simulink model "HILModel"  (R2016a)
settings: Solver=ode23tb  StartTime=0.0  StopTime=1000  RelTol=1e-3
libraries: DAEMOT_Lib x52
settings Model: Creator=aksland2  LastModifiedBy=aksland2

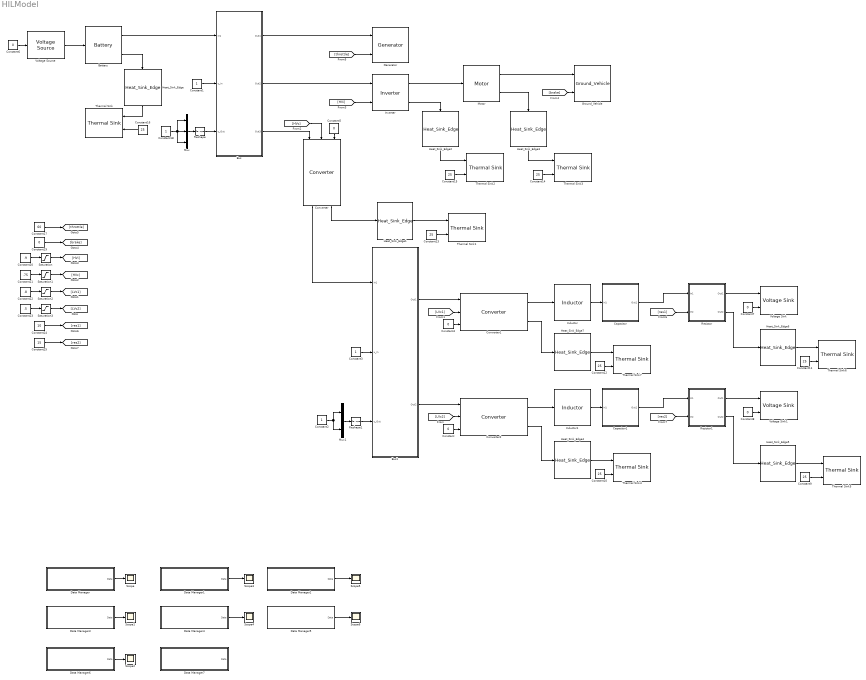
== system HILModel ==
  Battery : DAEMOT_Lib/Dyn Electrical Comp/Battery  C_c=62.7  C_s=4.5  R_cond=1.94  B_cap=5.088600000000000  Ns=16  Np=1  batt=4.2V LiPo 5.1 Ah  Ts_initial=25  Tc_initial=25  SOC_initial=.9  RC_initial=[0 0]
  Bus : Subsystem  AncestorBlock=DAEMOT_Lib/Electrical Components Chris/Bus  mask{R=.1, L=.0001, C=1, Num_In=1, Num_Out=3, V_initial=.5, I_initial=0}
      mask prompts: R "Resistance [Ohm]"; L "Inductance [H]"; C "Capacitance [F]"; Num_In "Number of Inputs"; Num_Out "Number of Outputs"; V_initial "Initial Voltage [V]"; I_initial "Initial Current [A]"
      mask init:
      | h      = get_param(gcb,'handle');   % Get block handle
      | blk    = gcb;
      | hblock = get(h);     % Parse out handles structure
      | 
      | %%%%%%%%%%%%%%%%%%%%%%%%%%%%%% Clear Stuff %%%%%%%%%%%%%%%%%%%%%%%%%%%%%%%%
      | %delete any previous inports and bus selectors
      | for i = str2num(hblock.Num_In)+1:hblock.Ports(1)-2
      |     delete_block([blk,'/In',num2str(i)])
      |     delete_block([blk,'/gb',num2str(i)])
      |     delete_block([blk,'/vm',num2str(i)])
      |     delete_block([blk,'/term',num2str(i)])
      |     delete_block([blk,'/Sink',num2str(i)])
      |     delete_block([blk,'/vin',num2str(i)])
      |     
      |     delete_unconnected_lines(blk)
      | end
      | 
      | for i = str2num(hblock.Num_Out)+1:hblock.Ports(2)
      |     delete_block([blk,'/Out',num2str(i)])
      |     delete_block([blk,'/if',num2str(i)])
      |     delete_block([blk,'/io',num2str(i)])
      |     delete_block([blk,'/vo',num2str(i)])
      |     delete_block([blk,'/vot',num2str(i)])
      |     delete_block([blk,'/b',num2str(i)])
      |     delete_block([blk,'/Source',num2str(i)])
      |     delete_block([blk,'/ig',num2str(i)])
      |     delete_block([blk,'/ios',num2str(i)])
      |     
      |     delete_unconnected_lines(blk)
      | end
      | %%%%%%%%%%%%%%%%%%%%%%%%%%%%% Clear Stuff %%%%%%%%%%%%%%%%%%%%%%%%%%%%%%%%
      | 
      | %%%%%%%%%%%%%%%%%%%%%%%%%%%%%% Edit Mux inputs %%%%%%%%%%%%%%%%%%%%%%%%%%%%%%%%
      | set_param([blk,'/Mux_In_1'],'Inputs',hblock.Num_In)
      | set_param([blk,'/Mux_In_2'],'Inputs',hblock.Num_Out)
      | set_param([blk,'/Demux_Out_1'],'Outputs',hblock.Num_In)
      | set_param([blk,'/Demux_Out_2'],'Outputs',hblock.Num_Out)
      | set_param([blk,'/u_Out'],'Port',num2str(Num_In+2))
      | set_param([blk,'/u_In'],'Port',num2str(Num_In+1))
      | set_param([blk,'/Bus_Sink_1'],'Inputs',num2str(str2num(hblock.Num_Out)+1))
      | 
      | %%%%%%%%%%%%%%%%%%%%%%%%%%%%%% Edit Mux inputs %%%%%%%%%%%%%%%%%%%%%%%%%%%%%%%%
      | 
      | %%%%%%%%%%%%%%%%%%%%%%%%%%%%%% Create and Place Inputs %%%%%%%%%%%%%%%%%%%%%%%%%%%%%%%%
      | % generate inports, bus selectors, and route lines to each vector concat
      | for i = hblock.Ports(1)+1-2:str2num(hblock.Num_In)
      |     
      |     % add blocks (positioning notation [x i*s+y x+l i*s+h+y] x:(horiz. pos.), y:(vert. pos.), s:(spacing), l:(horiz. length), x:(vert. height)
      |     add_block('simulink/Ports & Subsystems/In1',   [blk,'/In',num2str(i)],    'Position',[355 i*80+425 355+30 i*80+13+425]);         % adding inport
      |     add_block([blk,'/gb1'],                        [blk,'/gb',num2str(i)],   'Position',[440 i*80+410 440+5 i*80+38+410]);         % adding inport
      |     add_block('simulink/Signal Routing/Goto',      [blk,'/vm',num2str(i)],    'Position',[500 i*80+450 500+80 i*80+14+450]);         % adding inport
      |     add_block('simulink/Sinks/Terminator',          [blk,'/term',num2str(i)],    'Position',[500 i*80+415 500+20 i*80+14+415]);         % adding inport
      |     add_block('DAEMOT_Lib/Support Functions/Sink',[blk,'/Sink',num2str(i)],'Position',[200 i*30+336 200+65 i*30+28+336]);         % adding inport
      |     add_block('simulink/Signal Routing/From',       [blk,'/vin',num2str(i)],     'Position',[-400 i*20+405 -400+80 i*20+18+405]);         % adding inport
      |     
      |     % set goto and from tags
      |     set_param([blk,'/vm',num2str(i)],'GotoTag',char(horzcat('V_in',num2str(i))))
      |     set_param([blk,'/vin',num2str(i)],'GotoTag',char(horzcat('V_in',num2str(i))))
      |     
      |     % set goto and from background colors
      | %    set_param([blk,'/gm',num2str(i)],'BackgroundColor','yellow')
      | %    set_param([blk,'/gt',num2str(i)],'BackgroundColor','yellow')
      | %    %set_param([blk,'/gp',num2str(i)],'BackgroundColor','yellow')
      | %    set_param([blk,'/min',num2str(i)],'BackgroundColor','yellow')
      | %    set_param([blk,'/tin',num2str(i)],'BackgroundColor','yellow')
      | %    set_param([blk,'/pout',num2str(i)],'BackgroundColor','cyan')
      |     
      |     % add lines
      |     add_line(blk,['In',num2str(i),'/1'], ['gb',num2str(i),'/1'],'AutoRouting','on')
      |     add_line(blk,['gb',num2str(i),'/2'],  ['vm',num2str(i),'/1'],'AutoRouting','on')
      |     add_line(blk,['gb',num2str(i),'/1'],  ['term',num2str(i),'/1'],'AutoRouting','on')
      |     add_line(blk,['Demux_Out_1/',num2str(i)],  ['Sink',num2str(i),'/1'],'AutoRouting','on')
      |     add_line(blk,['vin',num2str(i),'/1'],  ['Mux_In_1/',num2str(i)],'AutoRouting','on')
      | %     
      | end
      | %%%%%%%%%%%%%%%%%%%%%%%%%%%%%% Create and Place Inputs %%%%%%%%%%%%%%%%%%%%%%%%%%%%%%%%
      | 
      | %%%%%%%%%%%%%%%%%%%%%%%%%%%%%% Create and Place Outputs %%%%%%%%%%%%%%%%%%%%%%%%%%%%%%%%
      | % generate inports, bus selectors, and route lines to each vector concat
      | for i = hblock.Ports(2)+1:str2num(hblock.Num_Out)
      |     
      |     % add blocks
      |     add_block('simulink/Ports & Subsystems/Out1',   [blk,'/Out',num2str(i)],   'Position',[875 i*80+425 875+30 i*80+13+425]);         % adding inport
      |     add_block('simulink/Signal Routing/Bus Creator',[blk,'/b',num2str(i)],     'Position',[825 i*80+410 825+5 i*80+38+410]);         % adding inport
      |     add_block('simulink/Signal Routing/From',       [blk,'/io',num2str(i)],     'Position',[710 i*80+415 710+80 i*80+14+415]);         % adding inport
      |     add_block('simulink/Signal Routing/From',       [blk,'/vo',num2str(i)],     'Position',[710 i*80+435 710+80 i*80+14+435]);         % adding inport
      |     add_block('simulink/Signal Routing/Goto',       [blk,'/vot',num2str(i)],     'Position',[1250 i*20+50 1250+80 i*20+18+50]);         % adding inport
      |     add_block('simulink/Signal Routing/From',       [blk,'/if',num2str(i)],     'Position',[935 i*20+410 935+80 i*20+18+410]);         % adding inport
      |     add_block('DAEMOT_Lib/Support Functions/Source',[blk,'/Source',num2str(i)],'Position',[1400 i*30+420 1400+65 i*30+28+420]);         % adding inport
      |     add_block('simulink/Signal Routing/Goto',       [blk,'/ig',num2str(i)],     'Position',[1550 i*30+430 1550+80 i*30+14+430]);         % adding inport
      |     add_block('simulink/Signal Routing/From',       [blk,'/ios',num2str(i)],     'Position',[1770 i*16+405 1770+80 i*16+14+405]);         % adding inport
      |     
      |     % set goto and from tags
      |     set_param([blk,'/if',num2str(i)],'GotoTag',char(horzcat('I_out',num2str(i))))
      |     set_param([blk,'/io',num2str(i)],'GotoTag',char(horzcat('I_out',num2str(i))))
      |     set_param([blk,'/vo',num2str(i)],'GotoTag',char(horzcat('V_out',num2str(i))))
      |     set_param([blk,'/vot',num2str(i)],'GotoTag',char(horzcat('V_out',num2str(i))))
      |     set_param([blk,'/ig',num2str(i)],'GotoTag',char(horzcat('I_out',num2str(i))))
      |     set_param([blk,'/ios',num2str(i)],'GotoTag',char(horzcat('I_out',num2str(i))))
      |     set_param([blk,'/b',num2str(i)],'Inputs','2')
      |     
      | %     % set goto and from background colors
      | %     set_param([blk,'/t',num2str(i)],'BackgroundColor','cyan')
      | %     set_param([blk,'/m',num2str(i)],'BackgroundColor','cyan')
      | %     set_param([blk,'/p',num2str(i)],'BackgroundColor','cyan')
      | %     set_param([blk,'/g',num2str(i)],'BackgroundColor','cyan')
      | %     set_param([blk,'/mout',num2str(i)],'BackgroundColor','cyan')
      | %     %set_param([blk,'/tout',num2str(i)],'BackgroundColor','cyan')
      |     
      |     % add lines
      |     add_line(blk,['io',num2str(i),'/1'],['b',num2str(i),'/1'],'AutoRouting','on')
      |     p = get_param([blk,'/io',num2str(i)],'PortHandles');
      |     l = get_param(p.Outport,'Line');
      |     set_param(l,'Name','current')
      |     
      |     add_line(blk,['vo',num2str(i),'/1'],['b',num2str(i),'/2'],'AutoRouting','on')
      |     p = get_param([blk,'/vo',num2str(i)],'PortHandles');
      |     l = get_param(p.Outport,'Line');
      |     set_param(l,'Name','voltage')
      |         
      |     add_line(blk,['ios',num2str(i),'/1'],['Bus_Sink_1/',num2str(i+1)],'AutoRouting','on')
      |     p = get_param([blk,'/ios',num2str(i)],'PortHandles');
      |     l = get_param(p.Outport,'Line');
      |     set_param(l,'Name',['Current',num2str(i)])
      |      
      |     add_line(blk,['b',num2str(i),'/1'],['Out',num2str(i),'/1'],'AutoRouting','on')
      |     add_line(blk,['Source',num2str(i),'/1'],['ig',num2str(i),'/1'],'AutoRouting','on')
      |     add_line(blk,['if',num2str(i),'/1'],  ['Mux_In_2/',num2str(i)],'AutoRouting','on')
      |     add_line(blk,['Demux_Out_2/',num2str(i)],['vot',num2str(i),'/1'],'AutoRouting','on')
      |     
      | 
      | 
      | end
      | %%%%%%%%%%%%%%%%%%%%%%%%%%%%%% Create and Place Outputs %%%%%%%%%%%%%%%%%%%%%%%%%%%%%%%%
      | 
      | try
      |     set_param([blk,'/Selector1'],'InputPortWidth',num2str(hblock.Num_In))
      |     
      |     selector_str = '[1 ';
      |     for i = 2:str2num(hblock.Num_In)
      |         selector_str = [selector_str,num2str(i),' '];
      |     end
      |     selector_str = [selector_str,']'];
      |     set_param([blk,'/Selector1'],'IndexParamArray',{selector_str})%num2cell(1:hblock.Num_In))
      | catch
      |     selector_str = '[1 ';
      |     for i = 2:str2num(hblock.Num_In)
      |         selector_str = [selector_str,num2str(i),' '];
      |     end
      |     selector_str = [selector_str,']'];
      |     set_param([blk,'/Selector1'],'IndexParamArray',{selector_str})%num2cell(1:hblock.Num_In))
      |     
      |     set_param([blk,'/Selector1'],'InputPortWidth',num2str(hblock.Num_In))
      | end 
      |     
      | try
      |     set_param([blk,'/Selector2'],'InputPortWidth',num2str(hblock.Num_Out))
      |     
      |     selector_str = '[1 ';
      |     for i = 2:str2num(hblock.Num_Out)
      |         selector_str = [selector_str,num2str(i),' '];
      |     end
      |     selector_str = [selector_str,']'];
      |     set_param([blk,'/Selector2'],'IndexParamArray',{selector_str})%num2cell(1:hblock.Num_Out))
      | catch
      |     selector_str = '[1 ';
      |     for i = 2:str2num(hblock.Num_Out)
      |         selector_str = [selector_str,num2str(i),' '];
      |     end
      |     selector_str = [selector_str,']'];
      |     set_param([blk,'/Selector2'],'IndexParamArray',{selector_str})%num2cell(1:hblock.Num_Out))
      |     
      |     set_param([blk,'/Selector2'],'InputPortWidth',num2str(hblock.Num_Out))
      | end 
      | 
      |     clear h blk hblock
      settings: CopyFcn=|
      | h      = get_param(gcb,'handle');   % Get block handle
      | blk    = gcb;
      | 
      | set_param(blk, 'LinkStatus', 'inactive')
      | clear h
      | clear blk
      mask Display:
      | text(0.5,0.95,['{\bf Bus}'],'TexMode','on','horizontalAlignment', 'center')
      | text(0.5,0.075,['{\bf ----(V)}'],'TexMode','on','horizontalAlignment', 'center')
      | 
      | In = get_param(gcb,'Num_In');
      | Out = get_param(gcb,'Num_Out');
      | 
      | for i = 1:str2num(In)
      |     port_label('input',i,['Electrical In ',num2str(i)])
      | end
      | 
      | port_label('input',str2num(In)+1,'u_In')
      | port_label('input',str2num(In)+2,'u_Out')
      | 
      | for i = 1:str2num(Out)
      |     port_label('output',i,['Electrical Out ',num2str(i)])
      | end
  Bus1 : Subsystem  AncestorBlock=DAEMOT_Lib/Electrical Components Chris/Bus  mask{R=.1, L=.0001, C=1, Num_In=1, Num_Out=2, V_initial=.5, I_initial=0}
      mask prompts: R "Resistance [Ohm]"; L "Inductance [H]"; C "Capacitance [F]"; Num_In "Number of Inputs"; Num_Out "Number of Outputs"; V_initial "Initial Voltage [V]"; I_initial "Initial Current [A]"
      mask init: same as HILModel/Bus
      settings: CopyFcn=|
      | h      = get_param(gcb,'handle');   % Get block handle
      | blk    = gcb;
      | 
      | set_param(blk, 'LinkStatus', 'inactive')
      | clear h
      | clear blk
      mask Display:
      | text(0.5,0.95,['{\bf Bus}'],'TexMode','on','horizontalAlignment', 'center')
      | text(0.5,0.075,['{\bf ----(V)}'],'TexMode','on','horizontalAlignment', 'center')
      | 
      | In = get_param(gcb,'Num_In');
      | Out = get_param(gcb,'Num_Out');
      | 
      | for i = 1:str2num(In)
      |     port_label('input',i,['Electrical In ',num2str(i)])
      | end
      | 
      | port_label('input',str2num(In)+1,'u_In')
      | port_label('input',str2num(In)+2,'u_Out')
      | 
      | for i = 1:str2num(Out)
      |     port_label('output',i,['Electrical Out ',num2str(i)])
      | end
  Capacitor : Subsystem  AncestorBlock=DAEMOT_Lib/Electrical Components Chris/Capacitor  mask{C=3, V_initial=0}
      mask prompts: C "Capacitance [F]"; V_initial "Initial Ouput Voltage [V]"
      mask init:
      | % if strcmp(Gn_check,'off')
      | %     %is not ground node
      | %     Gn = 0;
      | %     %V_initial = V_initial_temp;
      | % else
      | %     %is ground node
      | %     Gn = 1;
      | %     %V_initial = 0;
      | % end
      mask Display:
      | image(imread('capacitor.bmp'));
      | text(0.5,0.95,['{\bf Capacitor}'],'TexMode','on','horizontalAlignment', 'center')
      | text(0.5,0.075,['{\bf (V)}'],'TexMode','on','horizontalAlignment', 'center')
      | 
      | port_label('input',1,sprintf('Electrical \nIn'))
      | %port_label('input',2,'Capacitance')
      | port_label('output',1,sprintf('Electrical \nOut'))
  Capacitor1 : Subsystem  AncestorBlock=DAEMOT_Lib/Electrical Components Chris/Capacitor  mask{C=3, V_initial=0}
      mask prompts: C "Capacitance [F]"; V_initial "Initial Ouput Voltage [V]"
      mask init:
      | % if strcmp(Gn_check,'off')
      | %     %is not ground node
      | %     Gn = 0;
      | %     %V_initial = V_initial_temp;
      | % else
      | %     %is ground node
      | %     Gn = 1;
      | %     %V_initial = 0;
      | % end
      mask Display:
      | image(imread('capacitor.bmp'));
      | text(0.5,0.95,['{\bf Capacitor}'],'TexMode','on','horizontalAlignment', 'center')
      | text(0.5,0.075,['{\bf (V)}'],'TexMode','on','horizontalAlignment', 'center')
      | 
      | port_label('input',1,sprintf('Electrical \nIn'))
      | %port_label('input',2,'Capacitance')
      | port_label('output',1,sprintf('Electrical \nOut'))
  Constant{,4..8,19} (7 alike) : Constant  Value=0
  Constant{1..3,18} (4 alike) : Constant
  Constant{9..16} (8 alike) : Constant  Value=25
  Constant17 : Constant  Value=60
  Constant20 : Constant  Value=.9
  Constant21 : Constant  Value=.75
  Constant22 : Constant  Value=.8
  Constant23 : Constant  Value=.5
  Constant24 : Constant  Value=10
  Constant25 : Constant  Value=15
  Converter : DAEMOT_Lib/Dyn Electrical Comp/Converter  V_D=.01  R_D=.01  R_s=.01  R_L=.01  dir=<===  Cp=60  T_initial=25
  Converter1 : DAEMOT_Lib/Dyn Electrical Comp/Converter  V_D=.01  R_D=.01  R_s=.01  R_L=.01  dir=<===  Cp=60  T_initial=25
  Converter2 : DAEMOT_Lib/Dyn Electrical Comp/Converter  V_D=.01  R_D=.01  R_s=.01  R_L=.01  dir=<===  Cp=60  T_initial=25
  Data Manager : Subsystem  AncestorBlock=DAEMOT_Lib/Support Functions/Data Manager  mask{null=0}
      mask init:
      | set_param(gcb, 'LinkStatus', 'inactive')    % disable the library link
      settings: OpenFcn=data_manager
      mask Display: str ='Battery/SOC'; fprintf(str)
  Data Manager1 : Subsystem  AncestorBlock=DAEMOT_Lib/Support Functions/Data Manager  mask{null=0}
      mask init:
      | set_param(gcb, 'LinkStatus', 'inactive')    % disable the library link
      settings: OpenFcn=data_manager
      mask Display: str ='Bus/Voltage'; fprintf(str)
  Data Manager2 : Subsystem  AncestorBlock=DAEMOT_Lib/Support Functions/Data Manager  mask{null=0}
      mask init:
      | set_param(gcb, 'LinkStatus', 'inactive')    % disable the library link
      settings: OpenFcn=data_manager
      mask Display: str ='Bus1/Voltage'; fprintf(str)
  Data Manager3 : Subsystem  AncestorBlock=DAEMOT_Lib/Support Functions/Data Manager  mask{null=0}
      mask init:
      | set_param(gcb, 'LinkStatus', 'inactive')    % disable the library link
      settings: OpenFcn=data_manager
      mask Display: str ='Motor/Speed'; fprintf(str)
  Data Manager4 : Subsystem  AncestorBlock=DAEMOT_Lib/Support Functions/Data Manager  mask{null=0}
      mask init:
      | set_param(gcb, 'LinkStatus', 'inactive')    % disable the library link
      settings: OpenFcn=data_manager
      mask Display: str ='Ground_Vehicle/Vehicle Speed'; fprintf(str)
  Data Manager5 : Subsystem  AncestorBlock=DAEMOT_Lib/Support Functions/Data Manager  mask{null=0}
      mask init:
      | set_param(gcb, 'LinkStatus', 'inactive')    % disable the library link
      settings: OpenFcn=data_manager
      mask Display: str ='Generator/Current'; fprintf(str)
  Data Manager6 : Subsystem  AncestorBlock=DAEMOT_Lib/Support Functions/Data Manager  mask{null=0}
      mask init:
      | set_param(gcb, 'LinkStatus', 'inactive')    % disable the library link
      settings: OpenFcn=data_manager
      mask Display: str ='Resistor/Current\nResistor1/Current'; fprintf(str)
  Data Manager7 : Subsystem  AncestorBlock=DAEMOT_Lib/Support Functions/Data Manager  mask{null=0}
      mask init:
      | set_param(gcb, 'LinkStatus', 'inactive')    % disable the library link
      settings: OpenFcn=data_manager
      mask Display: str ='Ground_Vehicle/Vehicle Speed'; fprintf(str)
  Generator : DAEMOT_Lib/Dyn Electrical Comp/Generator  G=1
  Ground_Vehicle : DAEMOT_Lib/Dyn Electrical Comp/Ground_Vehicle  R=.3  Af=2  rho_air=1.2  Cd=.26
  Heat_Sink_Edge{,1..7} (8 alike) : DAEMOT_Lib/Dyn Electrical Comp/Heat_Sink_Edge  s=off  R_const=1  k=237  As=.025  L=.02
  Inductor : DAEMOT_Lib/Dyn Electrical Comp/Inductor  L=.0001  I_initial=0
  Inductor1 : DAEMOT_Lib/Dyn Electrical Comp/Inductor  L=.0001  I_initial=0
  Inverter : DAEMOT_Lib/Dyn Electrical Comp/Inverter  R1=.01  R2=.01  R3=.01  Cp=60  T_initial=25
  Motor : DAEMOT_Lib/Dyn Electrical Comp/Motor  R=0.013461960749493  L=1.252192537082724e-05  Kv=0.009688163543703  J=1.09*10^-4  b=1.89435163576232e-05  c=0.000234355495215172  GR=6.7  I_initial=1  w_initial=1  m_type=AC  Cp=60  T_initial=25
  Mux : Mux  Inputs=3
  Mux1 : Mux  Inputs=2
  Reshape : Reshape  OutputDimensionality=Column vector (2-D)
  Reshape1 : Reshape  OutputDimensionality=Column vector (2-D)
  Resistor : Subsystem  AncestorBlock=DAEMOT_Lib/Electrical Components Chris/Resistor  mask{r_type=Voltage, Cp=60, T_initial=25}
      mask prompts: r_type "Resistor Type"; Cp "Heat Capacity [J/K]"; T_initial "Initial Temperature [C]"
      mask init:
      | h      = get_param(gcb,'handle');   % Get block handle
      | blk    = gcb;
      | hblock = get(h);     % Parse out handles structure
      | 
      | if r_type == 1
      |     set_param([blk,'/From8'],'GotoTag',char('out'));
      |     set_param([blk,'/From10'],'GotoTag',char('in'));
      |     set_param([blk,'/From12'],'GotoTag',char('out'));
      |     set_param([blk,'/From4'],'GotoTag',char('out'));
      |     set_param([blk,'/From3'],'GotoTag',char('in'));
      | else
      |     set_param([blk,'/From8'],'GotoTag',char('in'));
      |     set_param([blk,'/From10'],'GotoTag',char('out'));
      |     set_param([blk,'/From12'],'GotoTag',char('in'));
      |     set_param([blk,'/From4'],'GotoTag',char('in'));
      |     set_param([blk,'/From3'],'GotoTag',char('out'));
      | end
      settings: CopyFcn=|
      | h      = get_param(gcb,'handle');   % Get block handle
      | blk    = gcb;
      | 
      | set_param(blk, 'LinkStatus', 'inactive')
      | clear h
      | clear blk
      mask TypeOptions r_type: Voltage | Current
      mask Display:
      | image(imread('resistor.bmp'));
      | T = get_param(gcb,'r_type');
      | text(0.5,0.95,['{\bf Resistor}'],'TexMode','on','horizontalAlignment', 'center')
      | if strcmp(T,'Current')
      |     text(0.5,0.075,['{\bf (V)*}'],'TexMode','on','horizontalAlignment', 'center')
      | else
      |     text(0.5,0.075,['{\bf ----}'],'TexMode','on','horizontalAlignment', 'center')
      | end
      | port_label('input',1,sprintf('Electrical \nIn'))
      | port_label('input',2,sprintf('Resistance \n[Ohm]'))
      | port_label('output',1,sprintf('Electrical \nOut'))
      | port_label('output',2,sprintf('Cooling \nOut'))
  Resistor1 : Subsystem  AncestorBlock=DAEMOT_Lib/Electrical Components Chris/Resistor  mask{r_type=Voltage, Cp=60, T_initial=25}
      mask prompts: r_type "Resistor Type"; Cp "Heat Capacity [J/K]"; T_initial "Initial Temperature [C]"
      mask init: same as HILModel/Resistor
      settings: CopyFcn=|
      | h      = get_param(gcb,'handle');   % Get block handle
      | blk    = gcb;
      | 
      | set_param(blk, 'LinkStatus', 'inactive')
      | clear h
      | clear blk
      mask TypeOptions r_type: Voltage | Current
      mask Display:
      | image(imread('resistor.bmp'));
      | T = get_param(gcb,'r_type');
      | text(0.5,0.95,['{\bf Resistor}'],'TexMode','on','horizontalAlignment', 'center')
      | if strcmp(T,'Current')
      |     text(0.5,0.075,['{\bf (V)*}'],'TexMode','on','horizontalAlignment', 'center')
      | else
      |     text(0.5,0.075,['{\bf ----}'],'TexMode','on','horizontalAlignment', 'center')
      | end
      | port_label('input',1,sprintf('Electrical \nIn'))
      | port_label('input',2,sprintf('Resistance \n[Ohm]'))
      | port_label('output',1,sprintf('Electrical \nOut'))
      | port_label('output',2,sprintf('Cooling \nOut'))
  Saturation{,1..3} (4 alike) : Saturate  UpperLimit=.99  LowerLimit=.01
  Scope{,1..6} (7 alike) : Scope
  Thermal Sink{,1..7} (8 alike) : DAEMOT_Lib/Dyn Electrical Comp/Sources and Sinks/Thermal Sink  M_ext=on  M=0  T_ext=on  T=0  P_ext=on  P=0
  Voltage Sink : DAEMOT_Lib/Dyn Electrical Comp/Sources and Sinks/Voltage Sink  M_ext=on  M=0  T_ext=on  T=0  P_ext=on  P=0
  Voltage Sink1 : DAEMOT_Lib/Dyn Electrical Comp/Sources and Sinks/Voltage Sink  M_ext=on  M=0  T_ext=on  T=0  P_ext=on  P=0
  Voltage Source : DAEMOT_Lib/Dyn Electrical Comp/Sources and Sinks/Voltage Source  M_ext=on  M=0  T_ext=on  T=0  P_ext=on  P=0
  wires:
  Battery/1 -> Bus/1(In1)
  Voltage Source/1 -> Battery/1
  Bus/1(Out1) -> Generator/1
  Bus/2(Out2) -> Inverter/1
  Inverter/1 -> Motor/1
  Motor/1 -> Ground_Vehicle/1
  Bus/3(Out3) -> Converter/1
  Converter/1 -> Bus1/1(In1)
  Bus1/1(Out1) -> Converter1/1
  Bus1/2(Out2) -> Converter2/1
  Converter1/1 -> Inductor/1
  Inductor/1 -> Capacitor/1(In1)
  Converter2/1 -> Inductor1/1
  Capacitor/1(Out1) -> Resistor/1(In1)
  Resistor/1(Out1) -> Voltage Sink/1
  Resistor1/1(Out1) -> Voltage Sink1/1
  Mux1/1 -> Reshape1/1
  Constant2/1 -> Mux1/1, Mux1/2
  Reshape/1 -> Bus/3(u_Out)
  Mux/1 -> Reshape/1
  Constant18/1 -> Mux/2, Mux/1, Mux/3
  Reshape1/1 -> Bus1/3(u_Out)
  Constant1/1 -> Bus/2(u_In)
  Constant3/1 -> Bus1/2(u_In)
  Heat_Sink_Edge/1 -> Thermal Sink/1
  Converter/2 -> Heat_Sink_Edge1/1
  Heat_Sink_Edge1/1 -> Thermal Sink1/1
  Inverter/2 -> Heat_Sink_Edge2/1
  Heat_Sink_Edge2/1 -> Thermal Sink2/1
  Heat_Sink_Edge3/1 -> Thermal Sink3/1
  Motor/2 -> Heat_Sink_Edge3/1
  Heat_Sink_Edge4/1 -> Thermal Sink4/1
  Converter2/2 -> Heat_Sink_Edge4/1
  Heat_Sink_Edge5/1 -> Thermal Sink5/1
  Resistor1/2(Out2) -> Heat_Sink_Edge5/1
  Heat_Sink_Edge6/1 -> Thermal Sink6/1
  Resistor/2(Out2) -> Heat_Sink_Edge6/1
  Heat_Sink_Edge7/1 -> Thermal Sink7/1
  Converter1/2 -> Heat_Sink_Edge7/1
  Constant/1 -> Converter2/3
  Constant4/1 -> Converter1/3
  Constant5/1 -> Converter/3
  Constant6/1 -> Voltage Source/1
  Constant7/1 -> Voltage Sink/2
  Constant8/1 -> Voltage Sink1/2
  Constant9/1 -> Thermal Sink5/2
  Constant10/1 -> Thermal Sink4/2
  Constant11/1 -> Thermal Sink6/2
  Constant12/1 -> Thermal Sink7/2
  Constant13/1 -> Thermal Sink1/2
  Constant14/1 -> Thermal Sink3/2
  Constant15/1 -> Thermal Sink2/2
  Constant16/1 -> Thermal Sink/2
  [LVc2] -> Converter2/2
  [LVc1] -> Converter1/2
  [HVc] -> Converter/2
  [HVi] -> Inverter/2
  [brake] -> Ground_Vehicle/2
  [throttle] -> Generator/2
  [res1] -> Resistor/2(In2)
  [res2] -> Resistor1/2(In2)
  Constant17/1 -> [throttle]
  Constant19/1 -> [brake]
  Constant21/1 -> Saturation1/1
  Constant22/1 -> Saturation2/1
  Constant23/1 -> Saturation3/1
  Constant24/1 -> [res1]
  Constant25/1 -> [res2]
  Data Manager/1(Data) -> Scope/1
  Data Manager3/1(Data) -> Scope1/1
  Data Manager6/1(Data) -> Scope2/1
  Data Manager1/1(Data) -> Scope3/1
  Data Manager4/1(Data) -> Scope4/1
  Data Manager2/1(Data) -> Scope5/1
  Data Manager5/1(Data) -> Scope6/1
  Saturation/1 -> [HVi]
  Constant20/1 -> Saturation/1
  Saturation1/1 -> [HVc]
  Saturation2/1 -> [LVc1]
  Saturation3/1 -> [LVc2]
  Inductor1/1 -> Capacitor1/1(In1)
  Capacitor1/1(Out1) -> Resistor1/1(In1)
  Battery/2 -> Heat_Sink_Edge/1

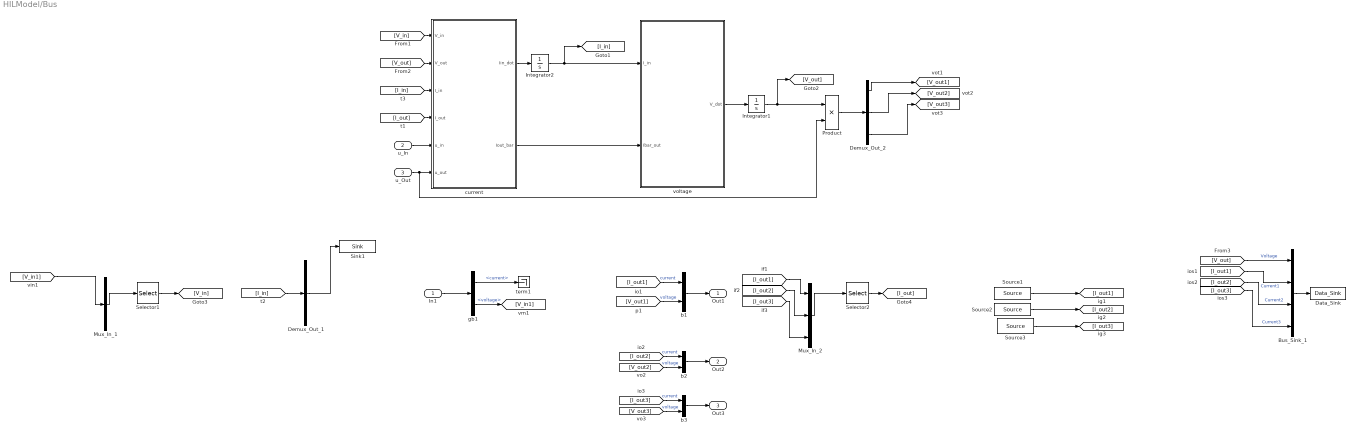
== system HILModel/Bus ==
  In1 : Inport
  u_In : Inport  Port=2
  u_Out : Inport  Port=3
  Bus_Sink_1 : BusCreator  Inputs=4
  Data_Sink : DAEMOT_Lib/Support Functions/Data_Sink
  Demux_Out_1 : Demux  Outputs=1
  Demux_Out_2 : Demux  Outputs=3
  Integrator1 : Integrator  InitialCondition=V_initial
  Integrator2 : Integrator  InitialCondition=I_initial*ones(Num_In,1)
  Mux_In_1 : Mux  Inputs=1
  Mux_In_2 : Mux  Inputs=3
  Product : Product
  Selector1 : Selector  InputPortWidth=1  IndexOptions=Index vector (dialog)  Indices=[1 ]  OutputSizes=1
  Selector2 : Selector  InputPortWidth=3  IndexOptions=Index vector (dialog)  Indices=[1 2 3 ]  OutputSizes=1
  Sink1 : DAEMOT_Lib/Support Functions/Sink
  Source1 : DAEMOT_Lib/Support Functions/Source
  Source2 : DAEMOT_Lib/Support Functions/Source
  Source3 : DAEMOT_Lib/Support Functions/Source
  b1 : BusCreator  Inputs=2
  b2 : BusCreator  Inputs=2
  b3 : BusCreator  Inputs=2
  current : MATLAB Function  TreatAsAtomicUnit=on
  gb1 : BusSelector  OutputSignals=current,voltage
  term1 : Terminator
  voltage : MATLAB Function  TreatAsAtomicUnit=on
  Out1 : Outport
  Out2 : Outport  Port=2
  Out3 : Outport  Port=3
  wires:
  Demux_Out_2/2 -> [V_out2]
  [I_out2] -> Mux_In_2/2
  Source2/1 -> [I_out2]
  b2/1 -> Out2/1
  [I_out2] -> Bus_Sink_1/3  "Current2"
  [V_out2] -> b2/2  "voltage"
  [I_out2] -> b2/1  "current"
  [I_out1] -> Bus_Sink_1/2  "Current1"
  [V_out] -> Bus_Sink_1/1  "Voltage"
  Selector2/1 -> [I_out]
  [I_out] -> current/4(I_out)
  Selector1/1 -> [V_in]
  [V_in] -> current/1(V_in)
  Product/1 -> Demux_Out_2/1
  current/2(Iout_bar) -> voltage/2(Ibar_out)
  u_Out/1 -> current/6(u_out), Product/2
  b1/1 -> Out1/1
  Source1/1 -> [I_out1]
  [I_out1] -> b1/1  "current"
  [V_out1] -> b1/2  "voltage"
  Mux_In_2/1 -> Selector2/1
  [I_out1] -> Mux_In_2/1
  Bus_Sink_1/1 -> Data_Sink/1
  Demux_Out_2/1 -> [V_out1]
  u_In/1 -> current/5(u_in)
  [I_in] -> current/3(I_in)
  current/1(Iin_dot) -> Integrator2/1
  Mux_In_1/1 -> Selector1/1
  [V_out] -> current/2(V_out)
  Integrator1/1 -> [V_out], Product/1
  voltage/1(V_dot) -> Integrator1/1
  Integrator2/1 -> [I_in], voltage/1(I_in)
  [I_in] -> Demux_Out_1/1
  In1/1 -> gb1/1
  gb1/1 -> term1/1  "<current>"
  gb1/2 -> [V_in1]  "<voltage>"
  [V_in1] -> Mux_In_1/1
  Demux_Out_1/1 -> Sink1/1
  [I_out3] -> b3/1  "current"
  [V_out3] -> b3/2  "voltage"
  [I_out3] -> Bus_Sink_1/4  "Current3"
  b3/1 -> Out3/1
  Source3/1 -> [I_out3]
  [I_out3] -> Mux_In_2/3
  Demux_Out_2/3 -> [V_out3]

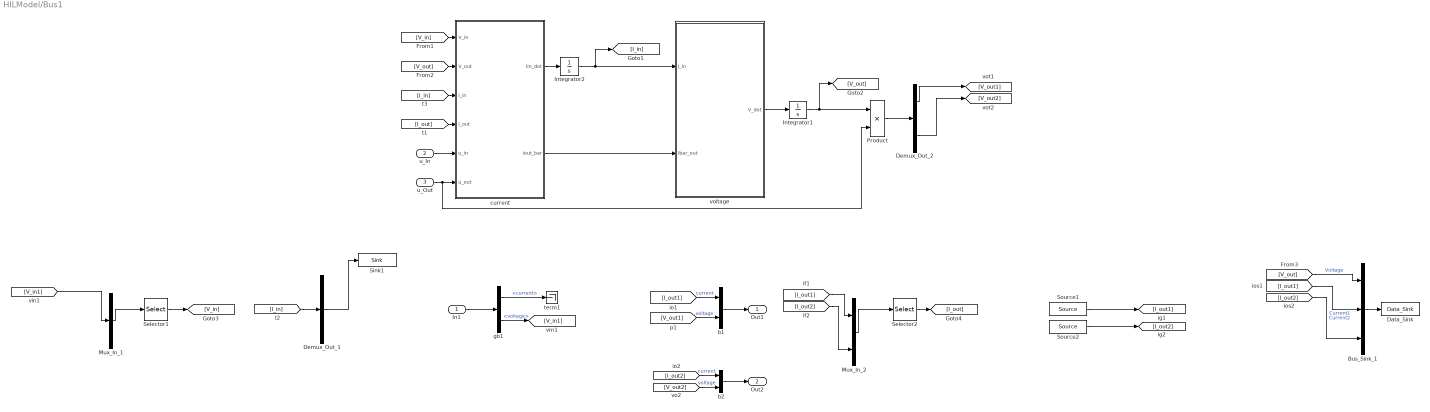
== system HILModel/Bus1 ==
  In1 : Inport
  u_In : Inport  Port=2
  u_Out : Inport  Port=3
  Bus_Sink_1 : BusCreator  Inputs=3
  Data_Sink : DAEMOT_Lib/Support Functions/Data_Sink
  Demux_Out_1 : Demux  Outputs=1
  Demux_Out_2 : Demux  Outputs=2
  Integrator1 : Integrator  InitialCondition=V_initial
  Integrator2 : Integrator  InitialCondition=I_initial*ones(Num_In,1)
  Mux_In_1 : Mux  Inputs=1
  Mux_In_2 : Mux  Inputs=2
  Product : Product
  Selector1 : Selector  InputPortWidth=1  IndexOptions=Index vector (dialog)  Indices=[1 ]  OutputSizes=1
  Selector2 : Selector  InputPortWidth=2  IndexOptions=Index vector (dialog)  Indices=[1 2 ]  OutputSizes=1
  Sink1 : DAEMOT_Lib/Support Functions/Sink
  Source1 : DAEMOT_Lib/Support Functions/Source
  Source2 : DAEMOT_Lib/Support Functions/Source
  b1 : BusCreator  Inputs=2
  b2 : BusCreator  Inputs=2
  current : MATLAB Function  TreatAsAtomicUnit=on
  gb1 : BusSelector  OutputSignals=current,voltage
  term1 : Terminator
  voltage : MATLAB Function  TreatAsAtomicUnit=on
  Out1 : Outport
  Out2 : Outport  Port=2
  wires:
  Demux_Out_1/1 -> Sink1/1
  [V_in1] -> Mux_In_1/1
  gb1/2 -> [V_in1]  "<voltage>"
  gb1/1 -> term1/1  "<current>"
  In1/1 -> gb1/1
  [I_in] -> Demux_Out_1/1
  Integrator2/1 -> voltage/1(I_in), [I_in]
  voltage/1(V_dot) -> Integrator1/1
  Integrator1/1 -> Product/1, [V_out]
  [V_out] -> current/2(V_out)
  Mux_In_1/1 -> Selector1/1
  current/1(Iin_dot) -> Integrator2/1
  [I_in] -> current/3(I_in)
  u_In/1 -> current/5(u_in)
  Demux_Out_2/1 -> [V_out1]
  Bus_Sink_1/1 -> Data_Sink/1
  [I_out1] -> Mux_In_2/1
  Mux_In_2/1 -> Selector2/1
  [V_out1] -> b1/2  "voltage"
  [I_out1] -> b1/1  "current"
  Source1/1 -> [I_out1]
  b1/1 -> Out1/1
  u_Out/1 -> Product/2, current/6(u_out)
  current/2(Iout_bar) -> voltage/2(Ibar_out)
  Product/1 -> Demux_Out_2/1
  [V_in] -> current/1(V_in)
  Selector1/1 -> [V_in]
  [I_out] -> current/4(I_out)
  Selector2/1 -> [I_out]
  [V_out] -> Bus_Sink_1/1  "Voltage"
  [I_out1] -> Bus_Sink_1/2  "Current1"
  [I_out2] -> b2/1  "current"
  [V_out2] -> b2/2  "voltage"
  [I_out2] -> Bus_Sink_1/3  "Current2"
  b2/1 -> Out2/1
  Source2/1 -> [I_out2]
  [I_out2] -> Mux_In_2/2
  Demux_Out_2/2 -> [V_out2]

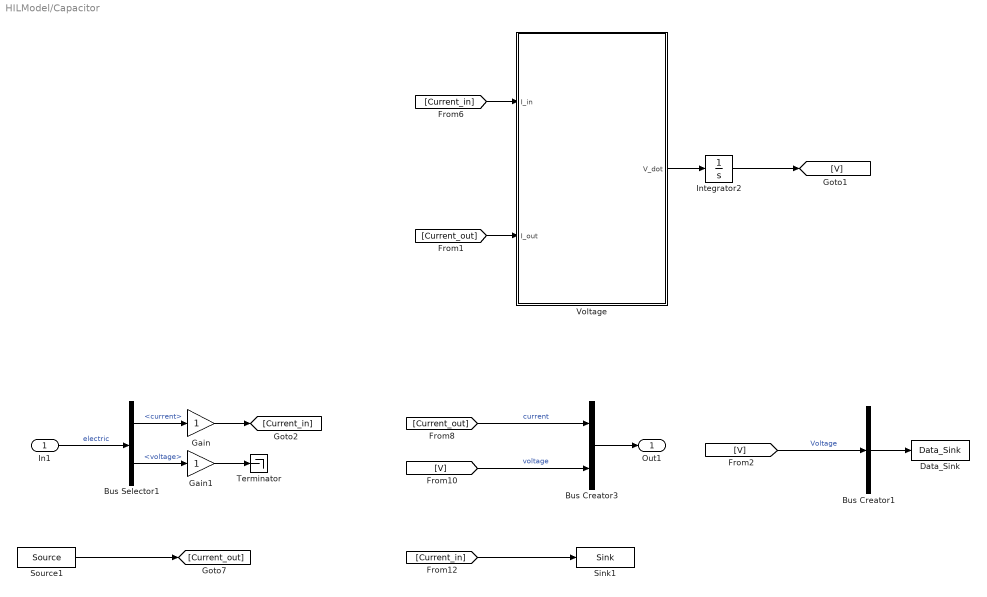
== system HILModel/Capacitor ==
  In1 : Inport
  Bus Creator1 : BusCreator  Inputs=1
  Bus Creator3 : BusCreator  Inputs=2
  Bus Selector1 : BusSelector  OutputSignals=current,voltage
  Data_Sink : DAEMOT_Lib/Support Functions/Data_Sink
  Gain : Gain
  Gain1 : Gain
  Integrator2 : Integrator  InitialCondition=V_initial
  Sink1 : DAEMOT_Lib/Support Functions/Sink
  Source1 : DAEMOT_Lib/Support Functions/Source
  Terminator : Terminator
  Voltage : MATLAB Function  TreatAsAtomicUnit=on
  Out1 : Outport
  wires:
  Gain1/1 -> Terminator/1
  Gain/1 -> [Current_in]
  Integrator2/1 -> [V]
  [Current_out] -> Bus Creator3/1  "current"
  Bus Selector1/1 -> Gain/1  "<current>"
  Bus Selector1/2 -> Gain1/1  "<voltage>"
  [V] -> Bus Creator3/2  "voltage"
  [Current_in] -> Sink1/1
  In1/1 -> Bus Selector1/1  "electric"
  [Current_out] -> Voltage/2(I_out)
  Bus Creator3/1 -> Out1/1
  Voltage/1(V_dot) -> Integrator2/1
  [Current_in] -> Voltage/1(I_in)
  [V] -> Bus Creator1/1  "Voltage"
  Bus Creator1/1 -> Data_Sink/1
  Source1/1 -> [Current_out]

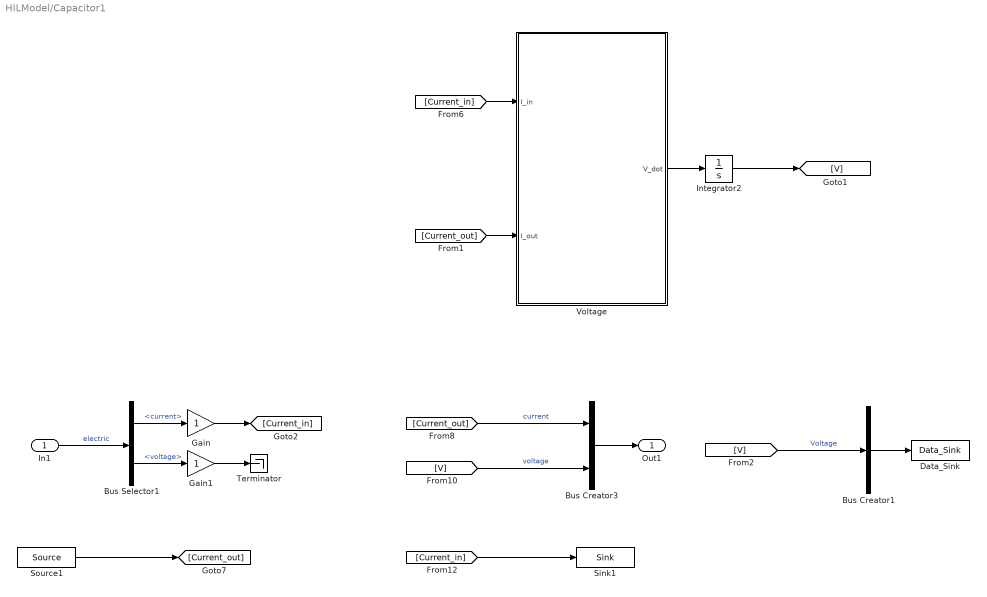
== system HILModel/Capacitor1 ==
  In1 : Inport
  Bus Creator1 : BusCreator  Inputs=1
  Bus Creator3 : BusCreator  Inputs=2
  Bus Selector1 : BusSelector  OutputSignals=current,voltage
  Data_Sink : DAEMOT_Lib/Support Functions/Data_Sink
  Gain : Gain
  Gain1 : Gain
  Integrator2 : Integrator  InitialCondition=V_initial
  Sink1 : DAEMOT_Lib/Support Functions/Sink
  Source1 : DAEMOT_Lib/Support Functions/Source
  Terminator : Terminator
  Voltage : MATLAB Function  TreatAsAtomicUnit=on
  Out1 : Outport
  wires:
  Source1/1 -> [Current_out]
  Bus Creator1/1 -> Data_Sink/1
  [V] -> Bus Creator1/1  "Voltage"
  [Current_in] -> Voltage/1(I_in)
  Voltage/1(V_dot) -> Integrator2/1
  Bus Creator3/1 -> Out1/1
  [Current_out] -> Voltage/2(I_out)
  In1/1 -> Bus Selector1/1  "electric"
  [Current_in] -> Sink1/1
  [V] -> Bus Creator3/2  "voltage"
  Bus Selector1/2 -> Gain1/1  "<voltage>"
  Bus Selector1/1 -> Gain/1  "<current>"
  [Current_out] -> Bus Creator3/1  "current"
  Integrator2/1 -> [V]
  Gain/1 -> [Current_in]
  Gain1/1 -> Terminator/1

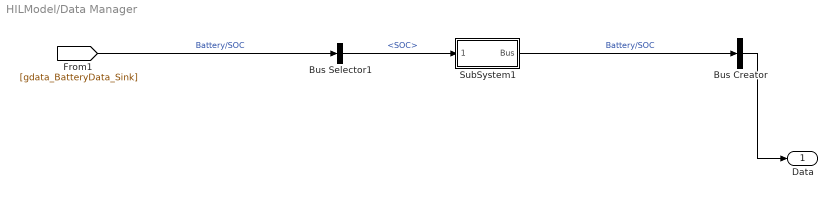
== system HILModel/Data Manager ==
  Bus Creator : BusCreator  Inputs=1
  Bus Selector1 : BusSelector  OutputSignals=SOC
  SubSystem1 : Subsystem
  Data : Outport
  wires:
  Bus Creator/1 -> Data/1
  [gdata_BatteryData_Sink] -> Bus Selector1/1  "Battery/SOC"
  Bus Selector1/1 -> SubSystem1/1(Rename)  "<SOC>"
  SubSystem1/1(Bus) -> Bus Creator/1  "Battery/SOC"

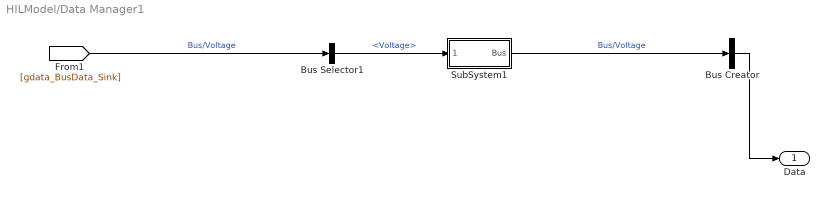
== system HILModel/Data Manager1 ==
  Bus Creator : BusCreator  Inputs=1
  Bus Selector1 : BusSelector  OutputSignals=Voltage
  SubSystem1 : Subsystem
  Data : Outport
  wires:
  Bus Creator/1 -> Data/1
  [gdata_BusData_Sink] -> Bus Selector1/1  "Bus/Voltage"
  Bus Selector1/1 -> SubSystem1/1(Rename)  "<Voltage>"
  SubSystem1/1(Bus) -> Bus Creator/1  "Bus/Voltage"

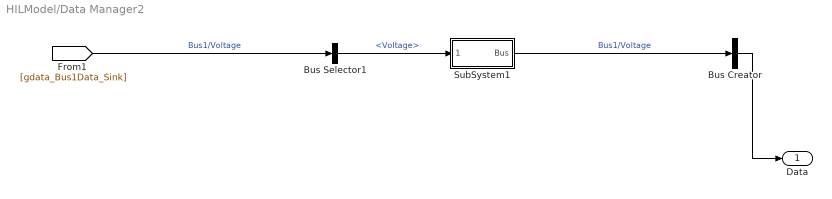
== system HILModel/Data Manager2 ==
  Bus Creator : BusCreator  Inputs=1
  Bus Selector1 : BusSelector  OutputSignals=Voltage
  SubSystem1 : Subsystem
  Data : Outport
  wires:
  Bus Creator/1 -> Data/1
  [gdata_Bus1Data_Sink] -> Bus Selector1/1  "Bus1/Voltage"
  Bus Selector1/1 -> SubSystem1/1(Rename)  "<Voltage>"
  SubSystem1/1(Bus) -> Bus Creator/1  "Bus1/Voltage"

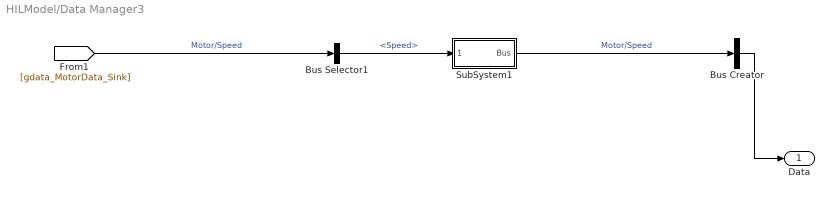
== system HILModel/Data Manager3 ==
  Bus Creator : BusCreator  Inputs=1
  Bus Selector1 : BusSelector  OutputSignals=Speed
  SubSystem1 : Subsystem
  Data : Outport
  wires:
  Bus Creator/1 -> Data/1
  [gdata_MotorData_Sink] -> Bus Selector1/1  "Motor/Speed"
  Bus Selector1/1 -> SubSystem1/1(Rename)  "<Speed>"
  SubSystem1/1(Bus) -> Bus Creator/1  "Motor/Speed"

== system HILModel/Data Manager4 ==
  Bus Creator : BusCreator  Inputs=1
  Bus Selector1 : BusSelector  OutputSignals=Vehicle Speed
  SubSystem1 : Subsystem
  Data : Outport
  wires:
  Bus Creator/1 -> Data/1
  [gdata_Ground_VehicleData_Sink] -> Bus Selector1/1  "Ground_Vehicle/Vehicle Speed"
  Bus Selector1/1 -> SubSystem1/1(Rename)  "<Vehicle Speed>"
  SubSystem1/1(Bus) -> Bus Creator/1  "Ground_Vehicle/Vehicle Speed"

== system HILModel/Data Manager5 ==
  Bus Creator : BusCreator  Inputs=1
  Bus Selector1 : BusSelector  OutputSignals=Current
  SubSystem1 : Subsystem
  Data : Outport
  wires:
  Bus Creator/1 -> Data/1
  [gdata_GeneratorData_Sink] -> Bus Selector1/1  "Generator/Current"
  Bus Selector1/1 -> SubSystem1/1(Rename)  "<Current>"
  SubSystem1/1(Bus) -> Bus Creator/1  "Generator/Current"

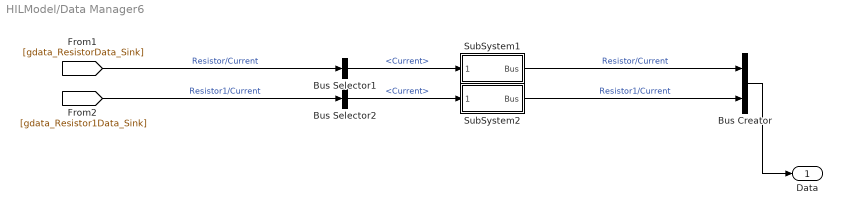
== system HILModel/Data Manager6 ==
  Bus Creator : BusCreator  Inputs=2
  Bus Selector1 : BusSelector  OutputSignals=Current
  Bus Selector2 : BusSelector  OutputSignals=Current
  SubSystem1 : Subsystem
  SubSystem2 : Subsystem
  Data : Outport
  wires:
  Bus Creator/1 -> Data/1
  [gdata_ResistorData_Sink] -> Bus Selector1/1  "Resistor/Current"
  Bus Selector1/1 -> SubSystem1/1(Rename)  "<Current>"
  SubSystem1/1(Bus) -> Bus Creator/1  "Resistor/Current"
  [gdata_Resistor1Data_Sink] -> Bus Selector2/1  "Resistor1/Current"
  Bus Selector2/1 -> SubSystem2/1(Rename)  "<Current>"
  SubSystem2/1(Bus) -> Bus Creator/2  "Resistor1/Current"

== system HILModel/Data Manager7 ==
  Bus Creator : BusCreator  Inputs=1
  Bus Selector1 : BusSelector  OutputSignals=Vehicle Speed
  SubSystem1 : Subsystem
  Data : Outport
  wires:
  SubSystem1/1(Bus) -> Bus Creator/1  "Ground_Vehicle/Vehicle Speed"
  Bus Selector1/1 -> SubSystem1/1(Rename)  "<Vehicle Speed>"
  [gdata_Ground_VehicleData_Sink] -> Bus Selector1/1  "Ground_Vehicle/Vehicle Speed"
  Bus Creator/1 -> Data/1

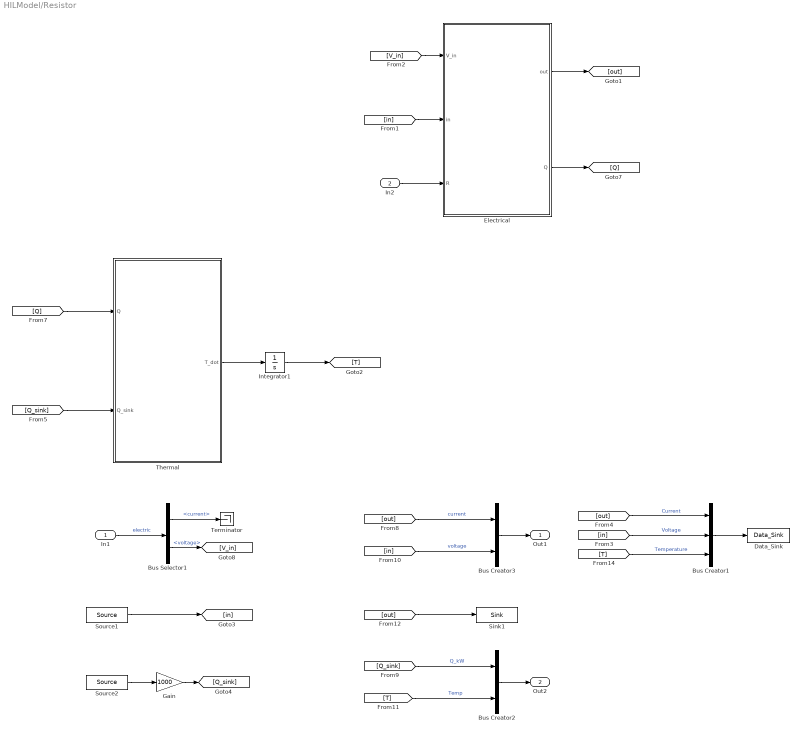
== system HILModel/Resistor ==
  In1 : Inport
  In2 : Inport  Port=2
  Bus Creator1 : BusCreator  Inputs=3
  Bus Creator2 : BusCreator  Inputs=2
  Bus Creator3 : BusCreator  Inputs=2
  Bus Selector1 : BusSelector  OutputSignals=current,voltage
  Data_Sink : DAEMOT_Lib/Support Functions/Data_Sink
  Electrical : MATLAB Function  TreatAsAtomicUnit=on
  Gain : Gain  Gain=1000
  Integrator1 : Integrator  InitialCondition=T_initial
  Sink1 : DAEMOT_Lib/Support Functions/Sink
  Source1 : DAEMOT_Lib/Support Functions/Source
  Source2 : DAEMOT_Lib/Support Functions/Source
  Terminator : Terminator
  Thermal : MATLAB Function  TreatAsAtomicUnit=on
  Out1 : Outport
  Out2 : Outport  Port=2
  wires:
  [Q_sink] -> Bus Creator2/1  "Q_kW"
  [T] -> Bus Creator2/2  "Temp"
  Bus Creator2/1 -> Out2/1
  [out] -> Bus Creator3/1  "current"
  Source1/1 -> [in]
  Bus Selector1/1 -> Terminator/1  "<current>"
  Bus Selector1/2 -> [V_in]  "<voltage>"
  [in] -> Bus Creator3/2  "voltage"
  [out] -> Sink1/1
  In1/1 -> Bus Selector1/1  "electric"
  Electrical/1(out) -> [out]
  Bus Creator3/1 -> Out1/1
  [V_in] -> Electrical/1(V_in)
  [in] -> Electrical/2(in)
  [out] -> Bus Creator1/1  "Current"
  [in] -> Bus Creator1/2  "Voltage"
  Bus Creator1/1 -> Data_Sink/1
  [Q_sink] -> Thermal/2(Q_sink)
  [Q] -> Thermal/1(Q)
  Integrator1/1 -> [T]
  Thermal/1(T_dot) -> Integrator1/1
  Electrical/2(Q) -> [Q]
  [T] -> Bus Creator1/3  "Temperature"
  Source2/1 -> Gain/1
  In2/1 -> Electrical/3(R)
  Gain/1 -> [Q_sink]

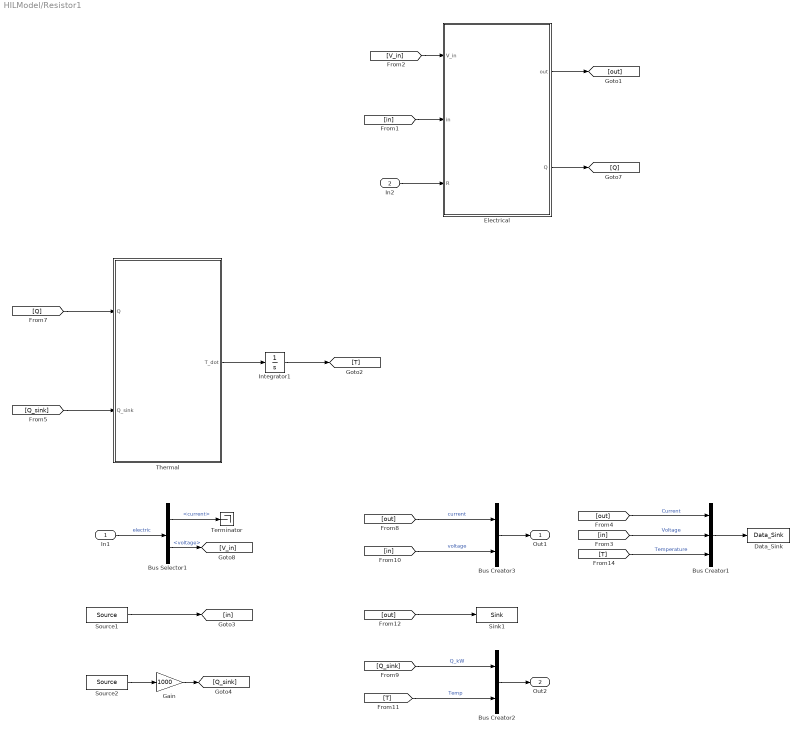
== system HILModel/Resistor1 ==
  In1 : Inport
  In2 : Inport  Port=2
  Bus Creator1 : BusCreator  Inputs=3
  Bus Creator2 : BusCreator  Inputs=2
  Bus Creator3 : BusCreator  Inputs=2
  Bus Selector1 : BusSelector  OutputSignals=current,voltage
  Data_Sink : DAEMOT_Lib/Support Functions/Data_Sink
  Electrical : MATLAB Function  TreatAsAtomicUnit=on
  Gain : Gain  Gain=1000
  Integrator1 : Integrator  InitialCondition=T_initial
  Sink1 : DAEMOT_Lib/Support Functions/Sink
  Source1 : DAEMOT_Lib/Support Functions/Source
  Source2 : DAEMOT_Lib/Support Functions/Source
  Terminator : Terminator
  Thermal : MATLAB Function  TreatAsAtomicUnit=on
  Out1 : Outport
  Out2 : Outport  Port=2
  wires:
  In2/1 -> Electrical/3(R)
  Source2/1 -> Gain/1
  [T] -> Bus Creator1/3  "Temperature"
  Electrical/2(Q) -> [Q]
  Thermal/1(T_dot) -> Integrator1/1
  Integrator1/1 -> [T]
  [Q] -> Thermal/1(Q)
  [Q_sink] -> Thermal/2(Q_sink)
  Bus Creator1/1 -> Data_Sink/1
  [in] -> Bus Creator1/2  "Voltage"
  [out] -> Bus Creator1/1  "Current"
  [in] -> Electrical/2(in)
  [V_in] -> Electrical/1(V_in)
  Bus Creator3/1 -> Out1/1
  Electrical/1(out) -> [out]
  In1/1 -> Bus Selector1/1  "electric"
  [out] -> Sink1/1
  [in] -> Bus Creator3/2  "voltage"
  Bus Selector1/2 -> [V_in]  "<voltage>"
  Bus Selector1/1 -> Terminator/1  "<current>"
  Source1/1 -> [in]
  [out] -> Bus Creator3/1  "current"
  Bus Creator2/1 -> Out2/1
  [T] -> Bus Creator2/2  "Temp"
  [Q_sink] -> Bus Creator2/1  "Q_kW"
  Gain/1 -> [Q_sink]

== system HILModel/Data Manager/SubSystem1 ==
  Rename : Inport
  Bus : Outport
  wires:
  Rename/1 -> Bus/1

== system HILModel/Data Manager1/SubSystem1 ==
  Rename : Inport
  Bus : Outport
  wires:
  Rename/1 -> Bus/1

== system HILModel/Data Manager2/SubSystem1 ==
  Rename : Inport
  Bus : Outport
  wires:
  Rename/1 -> Bus/1

== system HILModel/Data Manager3/SubSystem1 ==
  Rename : Inport
  Bus : Outport
  wires:
  Rename/1 -> Bus/1

== system HILModel/Data Manager4/SubSystem1 ==
  Rename : Inport
  Bus : Outport
  wires:
  Rename/1 -> Bus/1

== system HILModel/Data Manager5/SubSystem1 ==
  Rename : Inport
  Bus : Outport
  wires:
  Rename/1 -> Bus/1

== system HILModel/Data Manager6/SubSystem1 ==
  Rename : Inport
  Bus : Outport
  wires:
  Rename/1 -> Bus/1

== system HILModel/Data Manager6/SubSystem2 ==
  Rename : Inport
  Bus : Outport
  wires:
  Rename/1 -> Bus/1

== system HILModel/Data Manager7/SubSystem1 ==
  Rename : Inport
  Bus : Outport
  wires:
  Rename/1 -> Bus/1

== matlab function HILModel/Bus1/current ==
  data: Iin_dot output; V_in input; V_out input; I_in input; I_out input; u_in input; u_out input; L parameter; R parameter; Iout_bar output
function [Iin_dot,Iout_bar]= current(V_in,V_out,I_in,I_out,u_in,u_out, L,R)
%% Input Current

Iin_dot = (1/L) * ((V_in - V_out).*u_in - I_in*R);
Iout_bar = u_out'*I_out;

== matlab function HILModel/Bus1/voltage ==
  data: I_in input; Ibar_out input; V_dot output; C parameter
function V_dot = voltage(I_in,Ibar_out,C)
%% Output Voltage

Ibar_in = sum(I_in);
V_dot = (Ibar_in - Ibar_out)/C;

== matlab function HILModel/Resistor1/Electrical ==
  data: V_in input; out output; in input; R input; r_type parameter; Q output
function [out,Q]= voltage(V_in, in, R, r_type)
%% Output 

if r_type == 1 %voltage type
    out = (V_in - in)/R;
    Q = (V_in - in)/R^2;
else %current type
    out = V_in - in*R;
    Q = R^2*in;
end

== matlab function HILModel/Resistor1/Thermal ==
  data: Q input; T_dot output; Q_sink input; Cp parameter
function T_dot = Thermal(Q, Q_sink, Cp)
%% Load Temperature
T_dot = (1/Cp) * (Q - Q_sink);

== matlab function HILModel/Capacitor/Voltage ==
  data: I_in input; V_dot output; I_out input; C parameter
function V_dot = voltage(I_in, I_out,C)

V_dot = (1/C) * (I_in-I_out);

== matlab function HILModel/Capacitor1/Voltage ==
  data: I_in input; V_dot output; I_out input; C parameter
function V_dot = voltage(I_in, I_out,C)

V_dot = (1/C) * (I_in-I_out);

== matlab function HILModel/Resistor/Electrical ==
  data: V_in input; out output; in input; R input; r_type parameter; Q output
function [out,Q]= voltage(V_in, in, R, r_type)
%% Output 

if r_type == 1 %voltage type
    out = (V_in - in)/R;
    Q = (V_in - in)/R^2;
else %current type
    out = V_in - in*R;
    Q = R^2*in;
end

== matlab function HILModel/Resistor/Thermal ==
  data: Q input; T_dot output; Q_sink input; Cp parameter
function T_dot = Thermal(Q, Q_sink, Cp)
%% Load Temperature
T_dot = (1/Cp) * (Q - Q_sink);

== matlab function HILModel/Bus/current ==
  data: Iin_dot output; V_in input; V_out input; I_in input; I_out input; u_in input; u_out input; L parameter; R parameter; Iout_bar output
function [Iin_dot,Iout_bar]= current(V_in,V_out,I_in,I_out,u_in,u_out, L,R)
%% Input Current

Iin_dot = (1/L) * ((V_in - V_out).*u_in - I_in*R);
Iout_bar = u_out'*I_out;

== matlab function HILModel/Bus/voltage ==
  data: I_in input; Ibar_out input; V_dot output; C parameter
function V_dot = voltage(I_in,Ibar_out,C)
%% Output Voltage

Ibar_in = sum(I_in);
V_dot = (Ibar_in - Ibar_out)/C;
